simulink model "using_function_in_stateflow"  (R2020a)
settings: Solver=VariableStepAuto  StartTime=0.0  StopTime=10.0  RelTol=1e-3
settings Model: Creator=naina  LastModifiedBy=naina

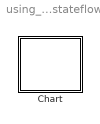
== system using_function_in_stateflow ==
  Chart : Stateflow chart  TreatAsAtomicUnit=on

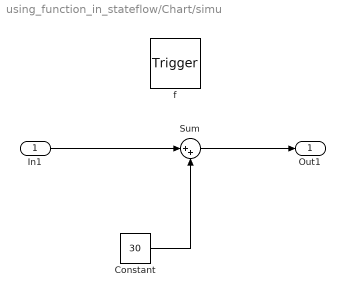
== system using_function_in_stateflow/Chart/simu ==
  In1 : Inport
  f : TriggerPort  TriggerType=function-call  VariantControl=(inherit)
      settings: CopyFcn=Stateflow.SLINSF.SimulinkMan.removeBlockPreDeleteFcn  PreDeleteFcn=Stateflow.SLINSF.SimulinkMan.unsafePredeleteFcn
  Constant : Constant  Value=30
  Sum : Sum  Inputs=|++
  Out1 : Outport
  wires:
  In1/1 -> Sum/1
  Sum/1 -> Out1/1
  Constant/1 -> Sum/2

== stateflow chart using_function_in_stateflow/Chart ==
  state A
  state B
    entry:
    x =3;
    y=simu(x);
  state Out1 = simu(In1) [function]
  state C
  (default) -> A
  A -> B : after(3,sec)
  B -> C : [u==3]
  data: In1 function_input; Out1 function_output
